simulink library "sm_boom_lift_crawler_lib_boom"  (R2026a)
settings: Solver=VariableStepAuto
undefined symbols (not defined in the file): B, b, BasketR, Extend, F, Jib, LevelM, LevelS, Lift, m, Tilt, Turret, X, Y, Z
libraries: sm_lib x228
(part 3 of 9)

== system sm_boom_lift_crawler_lib_boom/Boom/Turret/Case ==
  Bolts : sm_lib/Body Elements/File Solid  ExtGeomFileName=part243.step  UnitType=FromFile  ExtGeomFileUnits=m  StepReaderType=HEX  ExportConvexHullGeometry=off  InertiaType=CalculateFromGeometry  BasedOnType=Density  Density=rho.steel  DensityUnits=lbm/ft^3  Mass=1  MassUnits=kg  CenterOfMass=[0 0 0]  CenterOfMassUnits=m  MomentsOfInertia=[1 1 1]  MomentsOfInertiaUnits=kg*m^2  ProductsOfInertia=[0 0 0]  ProductsOfInertiaUnits=kg*m^2  GraphicType=FromGeometry  MarkerShape=Sphere  MarkerSize=10  GraphicVisPropType=AdvancedVisualProperties  GraphicDiffuseColor=rgb.metallic.c.diffuse  GraphicOpacity=1.0  GraphicSpecularColor=rgb.metallic.c.specular  GraphicAmbientColor=rgb.metallic.c.ambient  GraphicEmissiveColor=rgb.metallic.c.emissive  GraphicShininess=rgb.metallic.c.shininess  DoExposeReferenceFrame=on  SerializedFrames=<Frames/>
  Drive Case L : sm_lib/Body Elements/File Solid  ExtGeomFileName=part240.step  UnitType=FromFile  ExtGeomFileUnits=m  StepReaderType=HEX  ExportConvexHullGeometry=off  InertiaType=CalculateFromGeometry  BasedOnType=Density  Density=rho.aluminum  DensityUnits=lbm/ft^3  Mass=1  MassUnits=lbm  CenterOfMass=[0 0 0]  CenterOfMassUnits=in  MomentsOfInertia=[1 1 1]  MomentsOfInertiaUnits=lbm*in^2  ProductsOfInertia=[0 0 0]  ProductsOfInertiaUnits=lbm*in^2  GraphicType=FromGeometry  MarkerShape=Sphere  MarkerSize=10  GraphicVisPropType=AdvancedVisualProperties  GraphicDiffuseColor=rgb.metallic.a.diffuse  GraphicOpacity=1  GraphicSpecularColor=rgb.metallic.a.specular  GraphicAmbientColor=rgb.metallic.a.ambient  GraphicEmissiveColor=rgb.metallic.a.emissive  GraphicShininess=rgb.metallic.a.shininess  DoExposeReferenceFrame=on  SerializedFrames=<Frames><Frame><Id>Frame2</Id><Value><Name>F2</Name><Origin><Source>GeometricFeature</Source><FeatureName>circular curve 61</FeatureName></Origin><PrimaryAxis><DefinedDirection>-Z</DefinedDirection><Source>GeometricFeature</Source><SourceDirection>+Z</SourceDirection><FeatureName>circular curve 61</FeatureName></PrimaryAxis><SecondaryAxis><DefinedDirection>+X</DefinedDirection><Source>ReferenceFrame</Source><SourceDirection>+X</SourceDirection><FeatureName></FeatureName></SecondaryAxis></Value></Frame></Frames>
  Drive Case R : sm_lib/Body Elements/File Solid  ExtGeomFileName=part241.step  UnitType=FromFile  ExtGeomFileUnits=m  StepReaderType=HEX  ExportConvexHullGeometry=off  InertiaType=CalculateFromGeometry  BasedOnType=Density  Density=rho.aluminum  DensityUnits=lbm/ft^3  Mass=1  MassUnits=lbm  CenterOfMass=[0 0 0]  CenterOfMassUnits=in  MomentsOfInertia=[1 1 1]  MomentsOfInertiaUnits=lbm*in^2  ProductsOfInertia=[0 0 0]  ProductsOfInertiaUnits=lbm*in^2  GraphicType=FromGeometry  MarkerShape=Sphere  MarkerSize=10  GraphicVisPropType=AdvancedVisualProperties  GraphicDiffuseColor=rgb.metallic.a.diffuse  GraphicOpacity=1  GraphicSpecularColor=rgb.metallic.a.specular  GraphicAmbientColor=rgb.metallic.a.ambient  GraphicEmissiveColor=rgb.metallic.a.emissive  GraphicShininess=rgb.metallic.a.shininess  DoExposeReferenceFrame=on  SerializedFrames=<Frames><Frame><Id>Frame1</Id><Value><Name>F1</Name><Origin><Source>GeometricFeature</Source><FeatureName>circular curve 54</FeatureName></Origin><PrimaryAxis><DefinedDirection>+Z</DefinedDirection><Source>ReferenceFrame</Source><SourceDirection>+Z</SourceDirection><FeatureName></FeatureName></PrimaryAxis><SecondaryAxis><DefinedDirection>+X</DefinedDirection><Source>ReferenceFrame</Source><SourceDirection>+X</SourceDirection><FeatureName></FeatureName></SecondaryAxis></Value></Frame><Frame><Id>Frame2</Id><Value><Name>F2</Name><Origin><Source>GeometricFeature</Source><FeatureName>circular curve 55</FeatureName></Origin><PrimaryAxis><DefinedDirection>+Z</DefinedDirection><Source>ReferenceFrame</Source><SourceDirection>+Z</SourceDirection><FeatureName></FeatureName></PrimaryAxis><SecondaryAxis><DefinedDirection>+X</DefinedDirection><Source>ReferenceFrame</Source><SourceDirection>+X</SourceDirection><FeatureName></FeatureName></SecondaryAxis></Value></Frame></Frames>
  Free Wheel : sm_lib/Body Elements/File Solid  ExtGeomFileName=part242.step  UnitType=FromFile  ExtGeomFileUnits=m  StepReaderType=HEX  ExportConvexHullGeometry=off  InertiaType=CalculateFromGeometry  BasedOnType=Density  Density=rho.steel  DensityUnits=lbm/ft^3  Mass=1  MassUnits=lbm  CenterOfMass=[0 0 0]  CenterOfMassUnits=in  MomentsOfInertia=[1 1 1]  MomentsOfInertiaUnits=lbm*in^2  ProductsOfInertia=[0 0 0]  ProductsOfInertiaUnits=lbm*in^2  GraphicType=FromGeometry  MarkerShape=Sphere  MarkerSize=10  GraphicVisPropType=AdvancedVisualProperties  GraphicDiffuseColor=rgb.metallic.d.diffuse  GraphicOpacity=1  GraphicSpecularColor=rgb.metallic.d.specular  GraphicAmbientColor=rgb.metallic.d.ambient  GraphicEmissiveColor=rgb.metallic.d.emissive  GraphicShininess=rgb.metallic.d.shininess  DoExposeReferenceFrame=off  SerializedFrames=<Frames><Frame><Id>Frame1</Id><Value><Name>F1</Name><Origin><Source>GeometricFeature</Source><FeatureName>circular curve 60</FeatureName></Origin><PrimaryAxis><DefinedDirection>+Z</DefinedDirection><Source>ReferenceFrame</Source><SourceDirection>+Z</SourceDirection><FeatureName></FeatureName></PrimaryAxis><SecondaryAxis><DefinedDirection>+X</DefinedDirection><Source>ReferenceFrame</Source><SourceDirection>+X</SourceDirection><FeatureName></FeatureName></SecondaryAxis></Value></Frame><Frame><Id>Frame2</Id><Value><Name>F2</Name><Origin><Source>GeometricFeature</Source><FeatureName>toroidal surface 1</FeatureName></Origin><PrimaryAxis><DefinedDirection>+Z</DefinedDirection><Source>ReferenceFrame</Source><SourceDirection>+Z</SourceDirection><FeatureName></FeatureName></PrimaryAxis><SecondaryAxis><DefinedDirection>+X</DefinedDirection><Source>ReferenceFrame</Source><SourceDirection>+X</SourceDirection><FeatureName></FeatureName></SecondaryAxis></Value></Frame></Frames>
  Motor Cap : sm_lib/Body Elements/File Solid  ExtGeomFileName=part248.step  UnitType=FromFile  ExtGeomFileUnits=m  StepReaderType=HEX  ExportConvexHullGeometry=off  InertiaType=CalculateFromGeometry  BasedOnType=Density  Density=rho.aluminum  DensityUnits=lbm/ft^3  Mass=1  MassUnits=lbm  CenterOfMass=[0 0 0]  CenterOfMassUnits=in  MomentsOfInertia=[1 1 1]  MomentsOfInertiaUnits=lbm*in^2  ProductsOfInertia=[0 0 0]  ProductsOfInertiaUnits=lbm*in^2  GraphicType=FromGeometry  MarkerShape=Sphere  MarkerSize=10  GraphicVisPropType=AdvancedVisualProperties  GraphicDiffuseColor=rgb.metallic.e.diffuse  GraphicOpacity=1  GraphicSpecularColor=rgb.metallic.e.specular  GraphicAmbientColor=rgb.metallic.e.ambient  GraphicEmissiveColor=rgb.metallic.e.emissive  GraphicShininess=rgb.metallic.e.shininess  DoExposeReferenceFrame=on  SerializedFrames=<Frames/>
  Motor Case : sm_lib/Body Elements/File Solid  ExtGeomFileName=part244.step  UnitType=FromFile  ExtGeomFileUnits=m  StepReaderType=HEX  ExportConvexHullGeometry=off  InertiaType=CalculateFromGeometry  BasedOnType=Density  Density=rho.aluminum  DensityUnits=lbm/ft^3  Mass=1  MassUnits=lbm  CenterOfMass=[0 0 0]  CenterOfMassUnits=in  MomentsOfInertia=[1 1 1]  MomentsOfInertiaUnits=lbm*in^2  ProductsOfInertia=[0 0 0]  ProductsOfInertiaUnits=lbm*in^2  GraphicType=FromGeometry  MarkerShape=Sphere  MarkerSize=10  GraphicVisPropType=AdvancedVisualProperties  GraphicDiffuseColor=rgb.gray.e.diffuse  GraphicOpacity=1  GraphicSpecularColor=rgb.gray.e.specular  GraphicAmbientColor=rgb.gray.e.ambient  GraphicEmissiveColor=rgb.gray.e.emissive  GraphicShininess=rgb.gray.e.shininess  DoExposeReferenceFrame=off  SerializedFrames=<Frames><Frame><Id>Frame1</Id><Value><Name>F1</Name><Origin><Source>GeometricFeature</Source><FeatureName>circular curve 9</FeatureName></Origin><PrimaryAxis><DefinedDirection>-Z</DefinedDirection><Source>GeometricFeature</Source><SourceDirection>+Z</SourceDirection><FeatureName>circular curve 9</FeatureName></PrimaryAxis><SecondaryAxis><DefinedDirection>+X</DefinedDirection><Source>ReferenceFrame</Source><SourceDirection>+X</SourceDirection><FeatureName></FeatureName></SecondaryAxis></Value></Frame><Frame><Id>Frame2</Id><Value><Name>F2</Name><Origin><Source>GeometricFeature</Source><FeatureName>circular curve 9</FeatureName></Origin><PrimaryAxis><DefinedDirection>-Z</DefinedDirection><Source>GeometricFeature</Source><SourceDirection>+Z</SourceDirection><FeatureName>circular curve 9</FeatureName></PrimaryAxis><SecondaryAxis><DefinedDirection>+X</DefinedDirection><Source>ReferenceFrame</Source><SourceDirection>+X</SourceDirection><FeatureName></FeatureName></SecondaryAxis></Value></Frame></Frames>
  Reference Worm Cam : sm_lib/Frames and Transforms/Reference Frame
  Transform Worm Cam : sm_lib/Frames and Transforms/Rigid Transform  RotationMethod=RotationSequence  FollAlignAxisA=+X  BaseAlignAxisA=+Y  FollAlignAxisB=+Y  BaseAlignAxisB=+Z  RotationStandardAxis=+Z  RotationAngle=0.0  RotationAngleUnits=deg  RotationArbitraryAxis=[0 0 1]  RotationSequenceAxes=FollowerAxes  RotationSequence=YZY  RotationSequenceAngles=[-5 10 0]  RotationSequenceAnglesUnits=deg  RotationMatrix=[1 0 0; 0 1 0; 0 0 1]  Quaternion=[1 0 0 0]  TranslationMethod=Cartesian  TranslationCartesianOffset=[1 0.5 0.25]*(-0.25)  TranslationCartesianOffsetUnits=m  TranslationStandardAxis=+Z  TranslationStandardOffset=0  TranslationStandardOffsetUnits=m  TranslationROffset=0  TranslationROffsetUnits=m  TranslationThetaOffset=0  TranslationThetaOffsetUnits=deg  TranslationZOffset=0  TranslationZOffsetUnits=m
  Transforms : Subsystem
  F1 : PMIOPort  Side=Left
  F3 : PMIOPort  Port=2  Side=Right
  F2 : PMIOPort  Port=3  Side=Right
  connections:
  Transform Worm Cam/RConn1 -- Reference Worm Cam/RConn1
  Transform Worm Cam/LConn1 -- F1/RConn1 -- Transforms/RConn1
  F3/RConn1 -- Drive Case R/LConn2
  Drive Case L/LConn1 -- Motor Case/LConn1
  Free Wheel/RConn1 -- Transforms/LConn1 -- F2/RConn1
  Motor Cap/RConn1 -- Drive Case R/RConn1 -- Bolts/RConn1 -- Drive Case L/RConn1
  Drive Case R/LConn1 -- Free Wheel/LConn1

== system sm_boom_lift_crawler_lib_boom/Boom/Turret/Gear ==
  Bolts : sm_lib/Body Elements/File Solid  ExtGeomFileName=part247.step  UnitType=FromFile  ExtGeomFileUnits=m  StepReaderType=HEX  ExportConvexHullGeometry=off  InertiaType=CalculateFromGeometry  BasedOnType=Density  Density=rho.steel  DensityUnits=lbm/ft^3  Mass=1  MassUnits=kg  CenterOfMass=[0 0 0]  CenterOfMassUnits=m  MomentsOfInertia=[1 1 1]  MomentsOfInertiaUnits=kg*m^2  ProductsOfInertia=[0 0 0]  ProductsOfInertiaUnits=kg*m^2  GraphicType=FromGeometry  MarkerShape=Sphere  MarkerSize=10  GraphicVisPropType=AdvancedVisualProperties  GraphicDiffuseColor=rgb.metallic.c.diffuse  GraphicOpacity=1.0  GraphicSpecularColor=rgb.metallic.c.specular  GraphicAmbientColor=rgb.metallic.c.ambient  GraphicEmissiveColor=rgb.metallic.c.emissive  GraphicShininess=rgb.metallic.c.shininess  DoExposeReferenceFrame=on  SerializedFrames=<Frames/>
  Gear : sm_lib/Body Elements/File Solid  ExtGeomFileName=part245.step  UnitType=FromFile  ExtGeomFileUnits=m  StepReaderType=HEX  ExportConvexHullGeometry=off  InertiaType=CalculateFromGeometry  BasedOnType=Density  Density=rho.steel  DensityUnits=lbm/ft^3  Mass=1  MassUnits=kg  CenterOfMass=[0 0 0]  CenterOfMassUnits=m  MomentsOfInertia=[1 1 1]  MomentsOfInertiaUnits=kg*m^2  ProductsOfInertia=[0 0 0]  ProductsOfInertiaUnits=kg*m^2  GraphicType=FromGeometry  MarkerShape=Sphere  MarkerSize=10  GraphicVisPropType=AdvancedVisualProperties  GraphicDiffuseColor=rgb.metallic.f.diffuse  GraphicOpacity=1.0  GraphicSpecularColor=rgb.metallic.f.specular  GraphicAmbientColor=rgb.metallic.f.ambient  GraphicEmissiveColor=rgb.metallic.f.emissive  GraphicShininess=rgb.metallic.f.shininess  DoExposeReferenceFrame=on  SerializedFrames=<Frames><Frame><Id>Frame1</Id><Value><Name>F1</Name><Origin><Source>GeometricFeature</Source><FeatureName>toroidal surface 210</FeatureName></Origin><PrimaryAxis><DefinedDirection>+Z</DefinedDirection><Source>ReferenceFrame</Source><SourceDirection>+Z</SourceDirection><FeatureName></FeatureName></PrimaryAxis><SecondaryAxis><DefinedDirection>+X</DefinedDirection><Source>ReferenceFrame</Source><SourceDirection>+X</SourceDirection><FeatureName></FeatureName></SecondaryAxis></Value></Frame><Frame><Id>Frame2</Id><Value><Name>F2</Name><Origin><Source>GeometricFeature</Source><FeatureName>circular curve 523</FeatureName></Origin><PrimaryAxis><DefinedDirection>+Z</DefinedDirection><Source>ReferenceFrame</Source><SourceDirection>+Z</SourceDirection><FeatureName></FeatureName></PrimaryAxis><SecondaryAxis><DefinedDirection>+X</DefinedDirection><Source>ReferenceFrame</Source><SourceDirection>+X</SourceDirection><FeatureName></FeatureName></SecondaryAxis></Value></Frame></Frames>
  Rigid Transform : sm_lib/Frames and Transforms/Rigid Transform  RotationMethod=StandardAxis  FollAlignAxisA=+X  BaseAlignAxisA=+Y  FollAlignAxisB=+Y  BaseAlignAxisB=+Z  RotationStandardAxis=-Z  RotationAngle=45  RotationAngleUnits=deg  RotationArbitraryAxis=[0 0 1]  RotationSequenceAxes=FollowerAxes  RotationSequence=XYX  RotationSequenceAngles=[0 0 0]  RotationSequenceAnglesUnits=deg  RotationMatrix=[1 0 0; 0 1 0; 0 0 1]  Quaternion=[1 0 0 0]  TranslationMethod=None  TranslationCartesianOffset=[0 0 0]  TranslationCartesianOffsetUnits=m  TranslationStandardAxis=+Z  TranslationStandardOffset=0  TranslationStandardOffsetUnits=m  TranslationROffset=0  TranslationROffsetUnits=m  TranslationThetaOffset=0  TranslationThetaOffsetUnits=deg  TranslationZOffset=0  TranslationZOffsetUnits=m
  Seals : sm_lib/Body Elements/File Solid  ExtGeomFileName=part246.step  UnitType=FromFile  ExtGeomFileUnits=m  StepReaderType=HEX  ExportConvexHullGeometry=off  InertiaType=CalculateFromGeometry  BasedOnType=Density  Density=rho.steel  DensityUnits=lbm/ft^3  Mass=1  MassUnits=kg  CenterOfMass=[0 0 0]  CenterOfMassUnits=m  MomentsOfInertia=[1 1 1]  MomentsOfInertiaUnits=kg*m^2  ProductsOfInertia=[0 0 0]  ProductsOfInertiaUnits=kg*m^2  GraphicType=FromGeometry  MarkerShape=Sphere  MarkerSize=10  GraphicVisPropType=AdvancedVisualProperties  GraphicDiffuseColor=rgb.brights.red.diffuse  GraphicOpacity=1.0  GraphicSpecularColor=rgb.brights.red.specular  GraphicAmbientColor=rgb.brights.red.ambient  GraphicEmissiveColor=rgb.brights.red.emissive  GraphicShininess=rgb.brights.red.shininess  DoExposeReferenceFrame=on  SerializedFrames=<Frames/>
  F : PMIOPort  Side=Right
  F2 : PMIOPort  Port=2  Side=Right
  F1 : PMIOPort  Port=3  Side=Right
  connections:
  F1/RConn1 -- Rigid Transform/RConn1
  F2/RConn1 -- Gear/LConn2
  F/RConn1 -- Rigid Transform/LConn1 -- Gear/LConn1
  Gear/RConn1 -- Bolts/RConn1 -- Seals/RConn1

== system sm_boom_lift_crawler_lib_boom/Boom/Turret/Worm ==
  Worm : sm_lib/Body Elements/File Solid  ExtGeomFileName=part249.step  UnitType=FromFile  ExtGeomFileUnits=m  StepReaderType=HEX  ExportConvexHullGeometry=off  InertiaType=CalculateFromGeometry  BasedOnType=Density  Density=rho.steel  DensityUnits=lbm/ft^3  Mass=1  MassUnits=kg  CenterOfMass=[0 0 0]  CenterOfMassUnits=m  MomentsOfInertia=[1 1 1]  MomentsOfInertiaUnits=kg*m^2  ProductsOfInertia=[0 0 0]  ProductsOfInertiaUnits=kg*m^2  GraphicType=FromGeometry  MarkerShape=Sphere  MarkerSize=10  GraphicVisPropType=AdvancedVisualProperties  GraphicDiffuseColor=rgb.metallic.e.diffuse  GraphicOpacity=1.0  GraphicSpecularColor=rgb.metallic.e.specular  GraphicAmbientColor=rgb.metallic.e.ambient  GraphicEmissiveColor=rgb.metallic.e.emissive  GraphicShininess=rgb.metallic.e.shininess  DoExposeReferenceFrame=off  SerializedFrames=<Frames><Frame><Id>Frame1</Id><Value><Name>F1</Name><Origin><Source>GeometricFeature</Source><FeatureName>circular curve 4</FeatureName></Origin><PrimaryAxis><DefinedDirection>+Z</DefinedDirection><Source>GeometricFeature</Source><SourceDirection>+Z</SourceDirection><FeatureName>circular curve 4</FeatureName></PrimaryAxis><SecondaryAxis><DefinedDirection>+X</DefinedDirection><Source>ReferenceFrame</Source><SourceDirection>+X</SourceDirection><FeatureName></FeatureName></SecondaryAxis></Value></Frame><Frame><Id>Frame2</Id><Value><Name>F2</Name><Origin><Source>GeometricFeature</Source><FeatureName>cylindrical surface 3</FeatureName></Origin><PrimaryAxis><DefinedDirection>+Z</DefinedDirection><Source>GeometricFeature</Source><SourceDirection>+Z</SourceDirection><FeatureName>cylindrical surface 3</FeatureName></PrimaryAxis><SecondaryAxis><DefinedDirection>+X</DefinedDirection><Source>ReferenceFrame</Source><SourceDirection>+X</SourceDirection><FeatureName></FeatureName></SecondaryAxis></Value></Frame></Frames>
  F : PMIOPort  Side=Left
  F1 : PMIOPort  Port=2  Side=Right
  connections:
  Worm/RConn1 -- F/RConn1 -- F1/RConn1

== system sm_boom_lift_crawler_lib_boom/Boom/Arms/Basket Level Master Cylinder/Case ==
  Cap : sm_lib/Body Elements/File Solid  ExtGeomFileName=part170.step  UnitType=FromFile  ExtGeomFileUnits=m  StepReaderType=HEX  ExportConvexHullGeometry=off  InertiaType=CalculateFromGeometry  BasedOnType=Density  Density=rho.steel  DensityUnits=lbm/ft^3  Mass=1  MassUnits=lbm  CenterOfMass=[0 0 0]  CenterOfMassUnits=in  MomentsOfInertia=[1 1 1]  MomentsOfInertiaUnits=lbm*in^2  ProductsOfInertia=[0 0 0]  ProductsOfInertiaUnits=lbm*in^2  GraphicType=FromGeometry  MarkerShape=Sphere  MarkerSize=10  GraphicVisPropType=AdvancedVisualProperties  GraphicDiffuseColor=rgb.gray.b.diffuse  GraphicOpacity=1  GraphicSpecularColor=rgb.gray.b.specular  GraphicAmbientColor=rgb.gray.b.ambient  GraphicEmissiveColor=rgb.gray.b.emissive  GraphicShininess=rgb.gray.b.shininess  DoExposeReferenceFrame=off  SerializedFrames=<Frames><Frame><Id>Frame1</Id><Value><Name>F1</Name><Origin><Source>GeometricFeature</Source><FeatureName>circular curve 2</FeatureName></Origin><PrimaryAxis><DefinedDirection>+Z</DefinedDirection><Source>GeometricFeature</Source><SourceDirection>+Z</SourceDirection><FeatureName>circular curve 2</FeatureName></PrimaryAxis><SecondaryAxis><DefinedDirection>+X</DefinedDirection><Source>ReferenceFrame</Source><SourceDirection>+X</SourceDirection><FeatureName></FeatureName></SecondaryAxis></Value></Frame></Frames>
  Case : sm_lib/Body Elements/File Solid  ExtGeomFileName=part169.step  UnitType=FromFile  ExtGeomFileUnits=m  StepReaderType=HEX  ExportConvexHullGeometry=off  InertiaType=CalculateFromGeometry  BasedOnType=Density  Density=rho.steel  DensityUnits=lbm/ft^3  Mass=1  MassUnits=lbm  CenterOfMass=[0 0 0]  CenterOfMassUnits=in  MomentsOfInertia=[1 1 1]  MomentsOfInertiaUnits=lbm*in^2  ProductsOfInertia=[0 0 0]  ProductsOfInertiaUnits=lbm*in^2  GraphicType=FromGeometry  MarkerShape=Sphere  MarkerSize=10  GraphicVisPropType=AdvancedVisualProperties  GraphicDiffuseColor=rgb.gray.e.diffuse  GraphicOpacity=1  GraphicSpecularColor=rgb.gray.e.specular  GraphicAmbientColor=rgb.gray.e.ambient  GraphicEmissiveColor=rgb.gray.e.emissive  GraphicShininess=rgb.gray.e.shininess  DoExposeReferenceFrame=off  SerializedFrames=<Frames><Frame><Id>Frame1</Id><Value><Name>F1</Name><Origin><Source>GeometricFeature</Source><FeatureName>circular curve 16</FeatureName></Origin><PrimaryAxis><DefinedDirection>+Z</DefinedDirection><Source>ReferenceFrame</Source><SourceDirection>-X</SourceDirection><FeatureName></FeatureName></PrimaryAxis><SecondaryAxis><DefinedDirection>+Y</DefinedDirection><Source>ReferenceFrame</Source><SourceDirection>-Z</SourceDirection><FeatureName></FeatureName></SecondaryAxis></Value></Frame><Frame><Id>Frame2</Id><Value><Name>F2</Name><Origin><Source>GeometricFeature</Source><FeatureName>planar surface 7</FeatureName></Origin><PrimaryAxis><DefinedDirection>-Z</DefinedDirection><Source>GeometricFeature</Source><SourceDirection>+Z</SourceDirection><FeatureName>planar surface 7</FeatureName></PrimaryAxis><SecondaryAxis><DefinedDirection>+X</DefinedDirection><Source>ReferenceFrame</Source><SourceDirection>+X</SourceDirection><FeatureName></FeatureName></SecondaryAxis></Value></Frame><Frame><Id>Frame3</Id><Value><Name>F3</Name><Origin><Source>GeometricFeature</Source><FeatureName>circular curve 20</FeatureName></Origin><PrimaryAxis><DefinedDirection>-Z</DefinedDirection><Source>GeometricFeature</Source><SourceDirection>+Z</SourceDirection><FeatureName>circular curve 20</FeatureName></PrimaryAxis><SecondaryAxis><DefinedDirection>+X</DefinedDirection><Source>ReferenceFrame</Source><SourceDirection>+X</SourceDirection><FeatureName></FeatureName></SecondaryAxis></Value></Frame></Frames>
  F : PMIOPort  Side=Left
  F1 : PMIOPort  Port=2  Side=Right
  connections:
  Cap/LConn1 -- Case/LConn2
  F/RConn1 -- Case/RConn1
  F1/RConn1 -- Case/LConn1

== system sm_boom_lift_crawler_lib_boom/Boom/Arms/Basket Level Master Cylinder/Rod ==
  End : sm_lib/Body Elements/File Solid  ExtGeomFileName=part160.step  UnitType=FromFile  ExtGeomFileUnits=m  StepReaderType=HEX  ExportConvexHullGeometry=off  InertiaType=CalculateFromGeometry  BasedOnType=Density  Density=rho.steel  DensityUnits=lbm/ft^3  Mass=1  MassUnits=lbm  CenterOfMass=[0 0 0]  CenterOfMassUnits=in  MomentsOfInertia=[1 1 1]  MomentsOfInertiaUnits=lbm*in^2  ProductsOfInertia=[0 0 0]  ProductsOfInertiaUnits=lbm*in^2  GraphicType=FromGeometry  MarkerShape=Sphere  MarkerSize=10  GraphicVisPropType=AdvancedVisualProperties  GraphicDiffuseColor=rgb.gray.e.diffuse  GraphicOpacity=1  GraphicSpecularColor=rgb.gray.e.specular  GraphicAmbientColor=rgb.gray.e.ambient  GraphicEmissiveColor=rgb.gray.e.emissive  GraphicShininess=rgb.gray.e.shininess  DoExposeReferenceFrame=off  SerializedFrames=<Frames><Frame><Id>Frame1</Id><Value><Name>F1</Name><Origin><Source>GeometricFeature</Source><FeatureName>circular curve 2</FeatureName></Origin><PrimaryAxis><DefinedDirection>+Z</DefinedDirection><Source>GeometricFeature</Source><SourceDirection>+Z</SourceDirection><FeatureName>circular curve 3</FeatureName></PrimaryAxis><SecondaryAxis><DefinedDirection>+X</DefinedDirection><Source>ReferenceFrame</Source><SourceDirection>+X</SourceDirection><FeatureName></FeatureName></SecondaryAxis></Value></Frame><Frame><Id>Frame2</Id><Value><Name>F2</Name><Origin><Source>GeometricFeature</Source><FeatureName>circular curve 15</FeatureName></Origin><PrimaryAxis><DefinedDirection>-Z</DefinedDirection><Source>GeometricFeature</Source><SourceDirection>+Z</SourceDirection><FeatureName>circular curve 15</FeatureName></PrimaryAxis><SecondaryAxis><DefinedDirection>+Y</DefinedDirection><Source>ReferenceFrame</Source><SourceDirection>-Z</SourceDirection><FeatureName></FeatureName></SecondaryAxis></Value></Frame></Frames>
  Rod : sm_lib/Body Elements/File Solid  ExtGeomFileName=part161.step  UnitType=FromFile  ExtGeomFileUnits=m  StepReaderType=HEX  ExportConvexHullGeometry=off  InertiaType=CalculateFromGeometry  BasedOnType=Density  Density=rho.steel  DensityUnits=lbm/ft^3  Mass=1  MassUnits=lbm  CenterOfMass=[0 0 0]  CenterOfMassUnits=in  MomentsOfInertia=[1 1 1]  MomentsOfInertiaUnits=lbm*in^2  ProductsOfInertia=[0 0 0]  ProductsOfInertiaUnits=lbm*in^2  GraphicType=FromGeometry  MarkerShape=Sphere  MarkerSize=10  GraphicVisPropType=AdvancedVisualProperties  GraphicDiffuseColor=rgb.metallic.e.diffuse  GraphicOpacity=1  GraphicSpecularColor=rgb.metallic.e.specular  GraphicAmbientColor=rgb.metallic.e.ambient  GraphicEmissiveColor=rgb.metallic.e.emissive  GraphicShininess=rgb.metallic.e.shininess  DoExposeReferenceFrame=off  SerializedFrames=<Frames><Frame><Id>Frame1</Id><Value><Name>F1</Name><Origin><Source>GeometricFeature</Source><FeatureName>circular curve 2</FeatureName></Origin><PrimaryAxis><DefinedDirection>+Z</DefinedDirection><Source>GeometricFeature</Source><SourceDirection>+Z</SourceDirection><FeatureName>circular curve 2</FeatureName></PrimaryAxis><SecondaryAxis><DefinedDirection>+X</DefinedDirection><Source>ReferenceFrame</Source><SourceDirection>+X</SourceDirection><FeatureName></FeatureName></SecondaryAxis></Value></Frame><Frame><Id>Frame2</Id><Value><Name>F2</Name><Origin><Source>GeometricFeature</Source><FeatureName>circular curve 22</FeatureName></Origin><PrimaryAxis><DefinedDirection>-Z</DefinedDirection><Source>GeometricFeature</Source><SourceDirection>+Z</SourceDirection><FeatureName>circular curve 22</FeatureName></PrimaryAxis><SecondaryAxis><DefinedDirection>+X</DefinedDirection><Source>ReferenceFrame</Source><SourceDirection>+X</SourceDirection><FeatureName></FeatureName></SecondaryAxis></Value></Frame></Frames>
  F1 : PMIOPort  Side=Left
  F : PMIOPort  Port=2  Side=Right
  connections:
  Rod/LConn1 -- End/LConn1
  End/RConn1 -- F1/RConn1
  F/RConn1 -- Rod/RConn1

== system sm_boom_lift_crawler_lib_boom/Boom/Arms/Boom Tilt Cylinder/Case ==
  Cap : sm_lib/Body Elements/File Solid  ExtGeomFileName=part175.step  UnitType=FromFile  ExtGeomFileUnits=m  StepReaderType=HEX  ExportConvexHullGeometry=off  InertiaType=CalculateFromGeometry  BasedOnType=Density  Density=rho.steel  DensityUnits=lbm/ft^3  Mass=1  MassUnits=lbm  CenterOfMass=[0 0 0]  CenterOfMassUnits=in  MomentsOfInertia=[1 1 1]  MomentsOfInertiaUnits=lbm*in^2  ProductsOfInertia=[0 0 0]  ProductsOfInertiaUnits=lbm*in^2  GraphicType=FromGeometry  MarkerShape=Sphere  MarkerSize=10  GraphicVisPropType=AdvancedVisualProperties  GraphicDiffuseColor=rgb.gray.b.diffuse  GraphicOpacity=1  GraphicSpecularColor=rgb.gray.b.specular  GraphicAmbientColor=rgb.gray.b.ambient  GraphicEmissiveColor=rgb.gray.b.emissive  GraphicShininess=rgb.gray.b.shininess  DoExposeReferenceFrame=off  SerializedFrames=<Frames><Frame><Id>Frame1</Id><Value><Name>F1</Name><Origin><Source>GeometricFeature</Source><FeatureName>circular curve 1</FeatureName></Origin><PrimaryAxis><DefinedDirection>+Z</DefinedDirection><Source>GeometricFeature</Source><SourceDirection>+Z</SourceDirection><FeatureName>circular curve 1</FeatureName></PrimaryAxis><SecondaryAxis><DefinedDirection>+X</DefinedDirection><Source>ReferenceFrame</Source><SourceDirection>+Y</SourceDirection><FeatureName></FeatureName></SecondaryAxis></Value></Frame></Frames>
  Case : sm_lib/Body Elements/File Solid  ExtGeomFileName=part174.step  UnitType=FromFile  ExtGeomFileUnits=m  StepReaderType=HEX  ExportConvexHullGeometry=off  InertiaType=CalculateFromGeometry  BasedOnType=Density  Density=rho.steel  DensityUnits=lbm/ft^3  Mass=1  MassUnits=lbm  CenterOfMass=[0 0 0]  CenterOfMassUnits=in  MomentsOfInertia=[1 1 1]  MomentsOfInertiaUnits=lbm*in^2  ProductsOfInertia=[0 0 0]  ProductsOfInertiaUnits=lbm*in^2  GraphicType=FromGeometry  MarkerShape=Sphere  MarkerSize=10  GraphicVisPropType=AdvancedVisualProperties  GraphicDiffuseColor=rgb.gray.e.diffuse  GraphicOpacity=1  GraphicSpecularColor=rgb.gray.e.specular  GraphicAmbientColor=rgb.gray.e.ambient  GraphicEmissiveColor=rgb.gray.e.emissive  GraphicShininess=rgb.gray.e.shininess  DoExposeReferenceFrame=off  SerializedFrames=<Frames><Frame><Id>Frame1</Id><Value><Name>F1</Name><Origin><Source>GeometricFeature</Source><FeatureName>circular curve 2</FeatureName></Origin><PrimaryAxis><DefinedDirection>+Z</DefinedDirection><Source>ReferenceFrame</Source><SourceDirection>-X</SourceDirection><FeatureName></FeatureName></PrimaryAxis><SecondaryAxis><DefinedDirection>+Y</DefinedDirection><Source>ReferenceFrame</Source><SourceDirection>-Z</SourceDirection><FeatureName></FeatureName></SecondaryAxis></Value></Frame><Frame><Id>Frame2</Id><Value><Name>F2</Name><Origin><Source>GeometricFeature</Source><FeatureName>circular curve 13</FeatureName></Origin><PrimaryAxis><DefinedDirection>+Z</DefinedDirection><Source>GeometricFeature</Source><SourceDirection>+Z</SourceDirection><FeatureName>circular curve 13</FeatureName></PrimaryAxis><SecondaryAxis><DefinedDirection>+X</DefinedDirection><Source>ReferenceFrame</Source><SourceDirection>+X</SourceDirection><FeatureName></FeatureName></SecondaryAxis></Value></Frame><Frame><Id>Frame3</Id><Value><Name>F3</Name><Origin><Source>GeometricFeature</Source><FeatureName>circular curve 19</FeatureName></Origin><PrimaryAxis><DefinedDirection>-Z</DefinedDirection><Source>GeometricFeature</Source><SourceDirection>+Z</SourceDirection><FeatureName>planar surface 5</FeatureName></PrimaryAxis><SecondaryAxis><DefinedDirection>+X</DefinedDirection><Source>ReferenceFrame</Source><SourceDirection>+X</SourceDirection><FeatureName></FeatureName></SecondaryAxis></Value></Frame></Frames>
  F1 : PMIOPort  Side=Left
  F : PMIOPort  Port=2  Side=Right
  connections:
  F1/RConn1 -- Case/LConn2
  Cap/LConn1 -- Case/RConn1
  F/RConn1 -- Case/LConn1

== system sm_boom_lift_crawler_lib_boom/Boom/Arms/Boom Tilt Cylinder/Rod ==
  End : sm_lib/Body Elements/File Solid  ExtGeomFileName=part181.step  UnitType=FromFile  ExtGeomFileUnits=m  StepReaderType=HEX  ExportConvexHullGeometry=off  InertiaType=CalculateFromGeometry  BasedOnType=Density  Density=rho.steel  DensityUnits=lbm/ft^3  Mass=1  MassUnits=lbm  CenterOfMass=[0 0 0]  CenterOfMassUnits=in  MomentsOfInertia=[1 1 1]  MomentsOfInertiaUnits=lbm*in^2  ProductsOfInertia=[0 0 0]  ProductsOfInertiaUnits=lbm*in^2  GraphicType=FromGeometry  MarkerShape=Sphere  MarkerSize=10  GraphicVisPropType=AdvancedVisualProperties  GraphicDiffuseColor=rgb.gray.e.diffuse  GraphicOpacity=1  GraphicSpecularColor=rgb.gray.e.specular  GraphicAmbientColor=rgb.gray.e.ambient  GraphicEmissiveColor=rgb.gray.e.emissive  GraphicShininess=rgb.gray.e.shininess  DoExposeReferenceFrame=off  SerializedFrames=<Frames><Frame><Id>Frame1</Id><Value><Name>F1</Name><Origin><Source>GeometricFeature</Source><FeatureName>circular curve 6</FeatureName></Origin><PrimaryAxis><DefinedDirection>+Z</DefinedDirection><Source>ReferenceFrame</Source><SourceDirection>-X</SourceDirection><FeatureName></FeatureName></PrimaryAxis><SecondaryAxis><DefinedDirection>+Y</DefinedDirection><Source>ReferenceFrame</Source><SourceDirection>-Z</SourceDirection><FeatureName></FeatureName></SecondaryAxis></Value></Frame><Frame><Id>Frame2</Id><Value><Name>F2</Name><Origin><Source>GeometricFeature</Source><FeatureName>circular curve 1</FeatureName></Origin><PrimaryAxis><DefinedDirection>+Z</DefinedDirection><Source>GeometricFeature</Source><SourceDirection>+Z</SourceDirection><FeatureName>circular curve 1</FeatureName></PrimaryAxis><SecondaryAxis><DefinedDirection>+X</DefinedDirection><Source>ReferenceFrame</Source><SourceDirection>+X</SourceDirection><FeatureName></FeatureName></SecondaryAxis></Value></Frame></Frames>
  Rod : sm_lib/Body Elements/File Solid  ExtGeomFileName=part180.step  UnitType=FromFile  ExtGeomFileUnits=m  StepReaderType=HEX  ExportConvexHullGeometry=off  InertiaType=CalculateFromGeometry  BasedOnType=Density  Density=rho.steel  DensityUnits=lbm/ft^3  Mass=1  MassUnits=lbm  CenterOfMass=[0 0 0]  CenterOfMassUnits=in  MomentsOfInertia=[1 1 1]  MomentsOfInertiaUnits=lbm*in^2  ProductsOfInertia=[0 0 0]  ProductsOfInertiaUnits=lbm*in^2  GraphicType=FromGeometry  MarkerShape=Sphere  MarkerSize=10  GraphicVisPropType=AdvancedVisualProperties  GraphicDiffuseColor=rgb.metallic.e.diffuse  GraphicOpacity=1  GraphicSpecularColor=rgb.metallic.e.specular  GraphicAmbientColor=rgb.metallic.e.ambient  GraphicEmissiveColor=rgb.metallic.e.emissive  GraphicShininess=rgb.metallic.e.shininess  DoExposeReferenceFrame=off  SerializedFrames=<Frames><Frame><Id>Frame1</Id><Value><Name>F1</Name><Origin><Source>GeometricFeature</Source><FeatureName>circular curve 14</FeatureName></Origin><PrimaryAxis><DefinedDirection>-Z</DefinedDirection><Source>GeometricFeature</Source><SourceDirection>+Z</SourceDirection><FeatureName>circular curve 14</FeatureName></PrimaryAxis><SecondaryAxis><DefinedDirection>+X</DefinedDirection><Source>ReferenceFrame</Source><SourceDirection>+X</SourceDirection><FeatureName></FeatureName></SecondaryAxis></Value></Frame><Frame><Id>Frame2</Id><Value><Name>F2</Name><Origin><Source>GeometricFeature</Source><FeatureName>circular curve 1</FeatureName></Origin><PrimaryAxis><DefinedDirection>-Z</DefinedDirection><Source>GeometricFeature</Source><SourceDirection>+Z</SourceDirection><FeatureName>circular curve 1</FeatureName></PrimaryAxis><SecondaryAxis><DefinedDirection>+X</DefinedDirection><Source>ReferenceFrame</Source><SourceDirection>+X</SourceDirection><FeatureName></FeatureName></SecondaryAxis></Value></Frame></Frames>
  F1 : PMIOPort  Side=Right
  F : PMIOPort  Port=2  Side=Left
  connections:
  End/RConn1 -- Rod/RConn1
  F1/RConn1 -- Rod/LConn1
  F/RConn1 -- End/LConn1

== system sm_boom_lift_crawler_lib_boom/Boom/Arms/Telescope/Base Beam ==
  Base Left Half : Subsystem
      mask Display: image('sm041.svg')
  Base Right Half : Subsystem
      mask Display: image('sm040.svg')
  F6 : PMIOPort  Side=Right
  F : PMIOPort  Port=2  Side=Left
  F3 : PMIOPort  Port=3  Side=Left
  F2 : PMIOPort  Port=4  Side=Left
  F5 : PMIOPort  Port=5  Side=Right
  F8 : PMIOPort  Port=6  Side=Right
  F4 : PMIOPort  Port=7  Side=Left
  F10 : PMIOPort  Port=8  Side=Right
  F1 : PMIOPort  Port=9  Side=Right
  F7 : PMIOPort  Port=10  Side=Right
  connections:
  F5/RConn1 -- Base Right Half/LConn2
  F4/RConn1 -- Base Left Half/RConn5
  F3/RConn1 -- Base Left Half/RConn4
  F6/RConn1 -- Base Left Half/RConn2
  F1/RConn1 -- Base Left Half/LConn2
  F8/RConn1 -- Base Right Half/LConn1
  F2/RConn1 -- Base Left Half/RConn1
  F7/RConn1 -- Base Left Half/LConn1
  F/RConn1 -- Base Left Half/LConn4
  F10/RConn1 -- Base Left Half/LConn3
  Base Right Half/RConn1 -- Base Left Half/RConn3

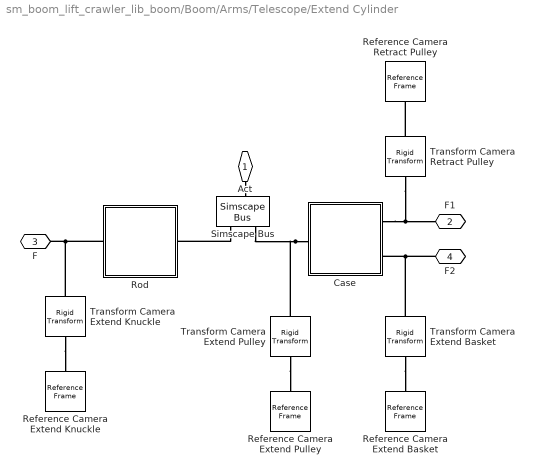
== system sm_boom_lift_crawler_lib_boom/Boom/Arms/Telescope/Extend Cylinder ==
  Case : Subsystem
  Reference Camera Extend Basket : sm_lib/Frames and Transforms/Reference Frame
  Reference Camera Extend Knuckle : sm_lib/Frames and Transforms/Reference Frame
  Reference Camera Extend Pulley : sm_lib/Frames and Transforms/Reference Frame
  Reference Camera Retract Pulley : sm_lib/Frames and Transforms/Reference Frame
  Rod : Subsystem
  Simscape Bus : SimscapeBus  HierarchyStrings=F;B
  Transform Camera Extend Basket : sm_lib/Frames and Transforms/Rigid Transform  RotationMethod=RotationSequence  FollAlignAxisA=+X  BaseAlignAxisA=+Y  FollAlignAxisB=+Y  BaseAlignAxisB=+Z  RotationStandardAxis=+Y  RotationAngle=35  RotationAngleUnits=deg  RotationArbitraryAxis=[0 0 1]  RotationSequenceAxes=FollowerAxes  RotationSequence=YZX  RotationSequenceAngles=[35 -20 0]  RotationSequenceAnglesUnits=deg  RotationMatrix=[1 0 0; 0 1 0; 0 0 1]  Quaternion=[1 0 0 0]  TranslationMethod=Cartesian  TranslationCartesianOffset=[-1 1 1.6]*0.7  TranslationCartesianOffsetUnits=m  TranslationStandardAxis=+Z  TranslationStandardOffset=0  TranslationStandardOffsetUnits=m  TranslationROffset=0  TranslationROffsetUnits=m  TranslationThetaOffset=0  TranslationThetaOffsetUnits=deg  TranslationZOffset=0  TranslationZOffsetUnits=m
  Transform Camera Extend Knuckle : sm_lib/Frames and Transforms/Rigid Transform  RotationMethod=StandardAxis  FollAlignAxisA=+X  BaseAlignAxisA=+Y  FollAlignAxisB=+Y  BaseAlignAxisB=+Z  RotationStandardAxis=+Y  RotationAngle=25  RotationAngleUnits=deg  RotationArbitraryAxis=[0 0 1]  RotationSequenceAxes=FollowerAxes  RotationSequence=XYX  RotationSequenceAngles=[0 0 0]  RotationSequenceAnglesUnits=deg  RotationMatrix=[1 0 0; 0 1 0; 0 0 1]  Quaternion=[1 0 0 0]  TranslationMethod=Cartesian  TranslationCartesianOffset=[0 0 -0.2]  TranslationCartesianOffsetUnits=m  TranslationStandardAxis=+Z  TranslationStandardOffset=0  TranslationStandardOffsetUnits=m  TranslationROffset=0  TranslationROffsetUnits=m  TranslationThetaOffset=0  TranslationThetaOffsetUnits=deg  TranslationZOffset=0  TranslationZOffsetUnits=m
  Transform Camera Extend Pulley : sm_lib/Frames and Transforms/Rigid Transform  RotationMethod=RotationSequence  FollAlignAxisA=+X  BaseAlignAxisA=+Y  FollAlignAxisB=+Y  BaseAlignAxisB=+Z  RotationStandardAxis=+Y  RotationAngle=35  RotationAngleUnits=deg  RotationArbitraryAxis=[0 0 1]  RotationSequenceAxes=FollowerAxes  RotationSequence=YZX  RotationSequenceAngles=[-30 0 0]  RotationSequenceAnglesUnits=deg  RotationMatrix=[1 0 0; 0 1 0; 0 0 1]  Quaternion=[1 0 0 0]  TranslationMethod=Cartesian  TranslationCartesianOffset=[1 0 -2]*0.4  TranslationCartesianOffsetUnits=m  TranslationStandardAxis=+Z  TranslationStandardOffset=0  TranslationStandardOffsetUnits=m  TranslationROffset=0  TranslationROffsetUnits=m  TranslationThetaOffset=0  TranslationThetaOffsetUnits=deg  TranslationZOffset=0  TranslationZOffsetUnits=m
  Transform Camera Retract Pulley : sm_lib/Frames and Transforms/Rigid Transform  RotationMethod=RotationSequence  FollAlignAxisA=+X  BaseAlignAxisA=+Y  FollAlignAxisB=+Y  BaseAlignAxisB=+Z  RotationStandardAxis=+Y  RotationAngle=35  RotationAngleUnits=deg  RotationArbitraryAxis=[0 0 1]  RotationSequenceAxes=FollowerAxes  RotationSequence=YZX  RotationSequenceAngles=[0 -30 0]  RotationSequenceAnglesUnits=deg  RotationMatrix=[1 0 0; 0 1 0; 0 0 1]  Quaternion=[1 0 0 0]  TranslationMethod=Cartesian  TranslationCartesianOffset=[-1 -1 0]*0.4  TranslationCartesianOffsetUnits=m  TranslationStandardAxis=+Z  TranslationStandardOffset=0  TranslationStandardOffsetUnits=m  TranslationROffset=0  TranslationROffsetUnits=m  TranslationThetaOffset=0  TranslationThetaOffsetUnits=deg  TranslationZOffset=0  TranslationZOffsetUnits=m
  Act : PMIOPort  Side=Left
  F1 : PMIOPort  Port=2  Side=Right
  F : PMIOPort  Port=3  Side=Right
  F2 : PMIOPort  Port=4  Side=Left
  connections:
  Transform Camera Extend Basket/RConn1 -- Reference Camera Extend Basket/RConn1
  Transform Camera Retract Pulley/RConn1 -- Reference Camera Retract Pulley/RConn1
  Act/RConn1 -- Simscape Bus/RConn1
  F2/RConn1 -- Transform Camera Extend Basket/LConn1 -- Case/LConn2
  Transform Camera Retract Pulley/LConn1 -- Case/LConn1 -- F1/RConn1
  Rod/RConn1 -- F/RConn1 -- Transform Camera Extend Knuckle/LConn1
  Simscape Bus/LConn1 -- Rod/LConn1
  Case/RConn1 -- Simscape Bus/LConn2 -- Transform Camera Extend Pulley/LConn1
  Transform Camera Extend Knuckle/RConn1 -- Reference Camera Extend Knuckle/RConn1
  Transform Camera Extend Pulley/RConn1 -- Reference Camera Extend Pulley/RConn1

== system sm_boom_lift_crawler_lib_boom/Boom/Arms/Telescope/Fly Beam ==
  Fly Left Half : Subsystem
      mask Display: image('sm045.svg')
  Fly Right Half : Subsystem
      mask Display: image('sm046.svg')
  F4 : PMIOPort  Side=Right
  F3 : PMIOPort  Port=2  Side=Right
  F1 : PMIOPort  Port=3  Side=Right
  F2 : PMIOPort  Port=4  Side=Right
  F : PMIOPort  Port=5  Side=Right
  F5 : PMIOPort  Port=6  Side=Right
  connections:
  Fly Left Half/RConn2 -- Fly Right Half/RConn1
  F5/RConn1 -- Fly Left Half/RConn1
  F3/RConn1 -- Fly Left Half/LConn2
  Fly Left Half/LConn1 -- F1/RConn1
  F/RConn1 -- Fly Right Half/RConn2
  F2/RConn1 -- Fly Right Half/LConn2
  F4/RConn1 -- Fly Right Half/LConn1

== system sm_boom_lift_crawler_lib_boom/Boom/Arms/Telescope/Middle Beam ==
  Cap : Subsystem
      mask Display: image('sm044.svg')
  Middle Left Half : Subsystem
      mask Display: image('sm043.svg')
  Middle Right Half : Subsystem
      mask Display: image('sm042.svg')
  Translation : sm_lib/Frames and Transforms/Rigid Transform  RotationMethod=None  FollAlignAxisA=+X  BaseAlignAxisA=+Y  FollAlignAxisB=+Y  BaseAlignAxisB=+Z  RotationStandardAxis=+Z  RotationAngle=0.0  RotationAngleUnits=deg  RotationArbitraryAxis=[0 0 1]  RotationSequenceAxes=FollowerAxes  RotationSequence=XYX  RotationSequenceAngles=[0 0 0]  RotationSequenceAnglesUnits=deg  RotationMatrix=[1 0 0; 0 1 0; 0 0 1]  Quaternion=[1 0 0 0]  TranslationMethod=Cartesian  TranslationCartesianOffset=[0 -0.5 6]  TranslationCartesianOffsetUnits=in  TranslationStandardAxis=-Y  TranslationStandardOffset=0.5  TranslationStandardOffsetUnits=in  TranslationROffset=0  TranslationROffsetUnits=m  TranslationThetaOffset=0  TranslationThetaOffsetUnits=deg  TranslationZOffset=0  TranslationZOffsetUnits=m
  F : PMIOPort  Side=Right
  F4 : PMIOPort  Port=2  Side=Left
  F3 : PMIOPort  Port=3  Side=Right
  F1 : PMIOPort  Port=4  Side=Left
  F5 : PMIOPort  Port=5  Side=Right
  connections:
  F5/RConn1 -- Middle Right Half/LConn2
  Translation/LConn1 -- Middle Right Half/LConn1
  F3/RConn1 -- Middle Left Half/LConn2
  F4/RConn1 -- Middle Left Half/LConn1
  F1/RConn1 -- Translation/RConn1
  Middle Left Half/RConn1 -- Middle Right Half/RConn1 -- Cap/LConn1
  Cap/RConn1 -- F/RConn1

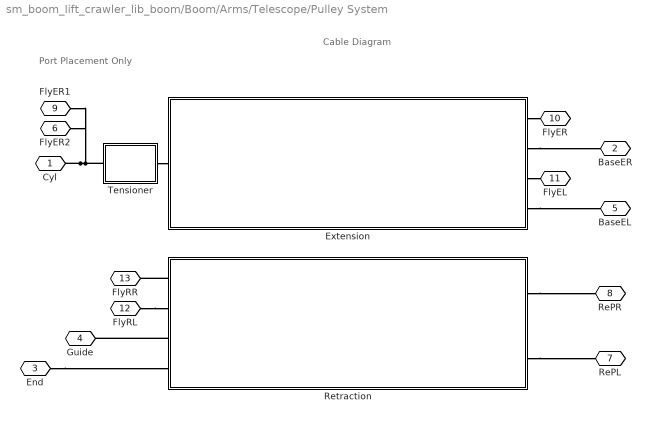
== system sm_boom_lift_crawler_lib_boom/Boom/Arms/Telescope/Pulley System ==
  note: Port
      | Placement
      | Only
  note: Cable Diagram
  Extension : Subsystem
      mask Display: image('sm_boom_lift_crawler_cable_extend_IMAGE.png');
  Retraction : Subsystem
      mask Display: image('sm_boom_lift_crawler_cable_retract_IMAGE.png')
  Tensioner : Subsystem  Variant=on  VariantControlMode=label  VariantControl=Variant1  LabelModeActiveChoice=On
  Cyl : PMIOPort  Side=Left
  BaseER : PMIOPort  Port=2  Side=Right
  End : PMIOPort  Port=3  Side=Right
  Guide : PMIOPort  Port=4  Side=Right
  BaseEL : PMIOPort  Port=5  Side=Right
  FlyER2 : PMIOPort  Port=6  Side=Right
  RePL : PMIOPort  Port=7  Side=Right
  RePR : PMIOPort  Port=8  Side=Right
  FlyER1 : PMIOPort  Port=9  Side=Right
  FlyER : PMIOPort  Port=10  Side=Right
  FlyEL : PMIOPort  Port=11  Side=Right
  FlyRL : PMIOPort  Port=12  Side=Right
  FlyRR : PMIOPort  Port=13  Side=Right
  connections:
  Tensioner/RConn1 -- Extension/LConn1
  Extension/RConn1 -- FlyER/RConn1
  Extension/RConn2 -- BaseER/RConn1
  FlyRL/RConn1 -- Retraction/LConn2
  Extension/RConn3 -- FlyEL/RConn1
  Extension/RConn4 -- BaseEL/RConn1
  Retraction/RConn1 -- RePR/RConn1
  Retraction/RConn2 -- RePL/RConn1
  Retraction/LConn1 -- FlyRR/RConn1
  End/RConn1 -- Retraction/LConn4
  Retraction/LConn3 -- Guide/RConn1
  Cyl/RConn1 -- Tensioner/LConn1 -- FlyER2/RConn1 -- FlyER1/RConn1

== system sm_boom_lift_crawler_lib_boom/Boom/Arms/Tower/Beam 1A ==
  Beam : sm_lib/Body Elements/File Solid  ExtGeomFileName=part043.step  UnitType=FromFile  ExtGeomFileUnits=m  StepReaderType=HEX  ExportConvexHullGeometry=off  InertiaType=CalculateFromGeometry  BasedOnType=Mass  Density=rho.steel  DensityUnits=lbm/ft^3  Mass=m.beam1A  MassUnits=lbm  CenterOfMass=[0 0 0]  CenterOfMassUnits=in  MomentsOfInertia=[1 1 1]  MomentsOfInertiaUnits=lbm*in^2  ProductsOfInertia=[0 0 0]  ProductsOfInertiaUnits=lbm*in^2  GraphicType=FromGeometry  MarkerShape=Sphere  MarkerSize=10  GraphicVisPropType=AdvancedVisualProperties  GraphicDiffuseColor=rgb.livery.b.diffuse  GraphicOpacity=1  GraphicSpecularColor=rgb.livery.b.specular  GraphicAmbientColor=rgb.livery.b.ambient  GraphicEmissiveColor=rgb.livery.b.emissive  GraphicShininess=rgb.livery.b.shininess  DoExposeReferenceFrame=off  SerializedFrames=<Frames><Frame><Id>Frame1</Id><Value><Name>F1</Name><Origin><Source>GeometricFeature</Source><FeatureName>circular curve 20</FeatureName></Origin><PrimaryAxis><DefinedDirection>+Z</DefinedDirection><Source>GeometricFeature</Source><SourceDirection>+Z</SourceDirection><FeatureName>circular curve 20</FeatureName></PrimaryAxis><SecondaryAxis><DefinedDirection>+X</DefinedDirection><Source>ReferenceFrame</Source><SourceDirection>+Y</SourceDirection><FeatureName></FeatureName></SecondaryAxis></Value></Frame><Frame><Id>Frame2</Id><Value><Name>F2</Name><Origin><Source>GeometricFeature</Source><FeatureName>circular curve 147</FeatureName></Origin><PrimaryAxis><DefinedDirection>+Z</DefinedDirection><Source>ReferenceFrame</Source><SourceDirection>-X</SourceDirection><FeatureName></FeatureName></PrimaryAxis><SecondaryAxis><DefinedDirection>+Y</DefinedDirection><Source>ReferenceFrame</Source><SourceDirection>+Z</SourceDirection><FeatureName></FeatureName></SecondaryAxis></Value></Frame><Frame><Id>Frame3</Id><Value><Name>F3</Name><Origin><Source>GeometricFeature</Source><FeatureName>circular curve 137</FeatureName></Origin><PrimaryAxis><DefinedDirection>+Z</DefinedDirection><Source>ReferenceFrame</Source><SourceDirection>-X</SourceDirection><FeatureName></FeatureName></PrimaryAxis><SecondaryAxis><DefinedDirection>+Y</DefinedDirection><Source>ReferenceFrame</Source><SourceDirection>-Z</SourceDirection><FeatureName></FeatureName></SecondaryAxis></Value></Frame></Frames>
  Hardware : Subsystem
  F3 : PMIOPort  Side=Left
  F1 : PMIOPort  Port=2  Side=Left
  F2 : PMIOPort  Port=3  Side=Right
  connections:
  F1/RConn1 -- Hardware/RConn2
  F3/RConn1 -- Beam/LConn2
  F2/RConn1 -- Beam/RConn1
  Hardware/RConn1 -- Beam/LConn1

== system sm_boom_lift_crawler_lib_boom/Boom/Arms/Tower/Beam 1B ==
  Beam : sm_lib/Body Elements/File Solid  ExtGeomFileName=part044.step  UnitType=FromFile  ExtGeomFileUnits=m  StepReaderType=HEX  ExportConvexHullGeometry=off  InertiaType=CalculateFromGeometry  BasedOnType=Mass  Density=rho.steel  DensityUnits=lbm/ft^3  Mass=m.beam1B  MassUnits=lbm  CenterOfMass=[0 0 0]  CenterOfMassUnits=in  MomentsOfInertia=[1 1 1]  MomentsOfInertiaUnits=lbm*in^2  ProductsOfInertia=[0 0 0]  ProductsOfInertiaUnits=lbm*in^2  GraphicType=FromGeometry  MarkerShape=Sphere  MarkerSize=10  GraphicVisPropType=AdvancedVisualProperties  GraphicDiffuseColor=rgb.livery.b.diffuse  GraphicOpacity=1  GraphicSpecularColor=rgb.livery.b.specular  GraphicAmbientColor=rgb.livery.b.ambient  GraphicEmissiveColor=rgb.livery.b.emissive  GraphicShininess=rgb.livery.b.shininess  DoExposeReferenceFrame=off  SerializedFrames=<Frames><Frame><Id>Frame1</Id><Value><Name>F1</Name><Origin><Source>GeometricFeature</Source><FeatureName>circular curve 214</FeatureName></Origin><PrimaryAxis><DefinedDirection>+Z</DefinedDirection><Source>ReferenceFrame</Source><SourceDirection>-X</SourceDirection><FeatureName></FeatureName></PrimaryAxis><SecondaryAxis><DefinedDirection>+Y</DefinedDirection><Source>ReferenceFrame</Source><SourceDirection>-Z</SourceDirection><FeatureName></FeatureName></SecondaryAxis></Value></Frame><Frame><Id>Frame2</Id><Value><Name>F2</Name><Origin><Source>GeometricFeature</Source><FeatureName>circular curve 32</FeatureName></Origin><PrimaryAxis><DefinedDirection>+Z</DefinedDirection><Source>ReferenceFrame</Source><SourceDirection>-X</SourceDirection><FeatureName></FeatureName></PrimaryAxis><SecondaryAxis><DefinedDirection>+Y</DefinedDirection><Source>ReferenceFrame</Source><SourceDirection>-Z</SourceDirection><FeatureName></FeatureName></SecondaryAxis></Value></Frame></Frames>
  F2 : PMIOPort  Side=Right
  F1 : PMIOPort  Port=2  Side=Left
  connections:
  F2/RConn1 -- Beam/RConn1
  F1/RConn1 -- Beam/LConn1

== system sm_boom_lift_crawler_lib_boom/Boom/Arms/Tower/Beam 2A1 ==
  Beam : sm_lib/Body Elements/File Solid  ExtGeomFileName=part048.step  UnitType=FromFile  ExtGeomFileUnits=m  StepReaderType=HEX  ExportConvexHullGeometry=off  InertiaType=CalculateFromGeometry  BasedOnType=Mass  Density=rho.steel  DensityUnits=lbm/ft^3  Mass=m.beam2A  MassUnits=lbm  CenterOfMass=[0 0 0]  CenterOfMassUnits=in  MomentsOfInertia=[1 1 1]  MomentsOfInertiaUnits=lbm*in^2  ProductsOfInertia=[0 0 0]  ProductsOfInertiaUnits=lbm*in^2  GraphicType=FromGeometry  MarkerShape=Sphere  MarkerSize=10  GraphicVisPropType=AdvancedVisualProperties  GraphicDiffuseColor=rgb.livery.b.diffuse  GraphicOpacity=1  GraphicSpecularColor=rgb.livery.b.specular  GraphicAmbientColor=rgb.livery.b.ambient  GraphicEmissiveColor=rgb.livery.b.emissive  GraphicShininess=rgb.livery.b.shininess  DoExposeReferenceFrame=off  SerializedFrames=<Frames><Frame><Id>Frame1</Id><Value><Name>F1</Name><Origin><Source>GeometricFeature</Source><FeatureName>circular curve 11</FeatureName></Origin><PrimaryAxis><DefinedDirection>+Z</DefinedDirection><Source>ReferenceFrame</Source><SourceDirection>-X</SourceDirection><FeatureName></FeatureName></PrimaryAxis><SecondaryAxis><DefinedDirection>+Y</DefinedDirection><Source>ReferenceFrame</Source><SourceDirection>-Z</SourceDirection><FeatureName></FeatureName></SecondaryAxis></Value></Frame><Frame><Id>Frame2</Id><Value><Name>F2</Name><Origin><Source>GeometricFeature</Source><FeatureName>circular curve 31</FeatureName></Origin><PrimaryAxis><DefinedDirection>+Z</DefinedDirection><Source>ReferenceFrame</Source><SourceDirection>-X</SourceDirection><FeatureName></FeatureName></PrimaryAxis><SecondaryAxis><DefinedDirection>+Y</DefinedDirection><Source>ReferenceFrame</Source><SourceDirection>-Z</SourceDirection><FeatureName></FeatureName></SecondaryAxis></Value></Frame></Frames>
  F1 : PMIOPort  Side=Left
  F : PMIOPort  Port=2  Side=Right
  connections:
  F1/RConn1 -- Beam/RConn1
  F/RConn1 -- Beam/LConn1
